simulink model "update_perfil_obstaculos_test"  (R2019a)
settings: Solver=VariableStepAuto  StartTime=0.0  StopTime=10  RelTol=1e-3
undefined symbols (not defined in the file): H_c, x_t_max_oper, x_t_min_oper, y_h_min_oper
libraries: simulink x1
settings Model: Creator=Facundo  LastModifiedBy=Facundo

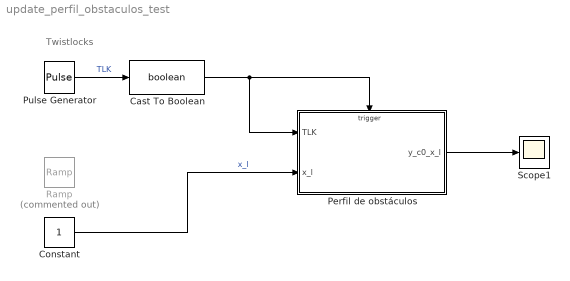
== system update_perfil_obstaculos_test ==
  note: Twistlocks
  Cast To Boolean : DataTypeConversion  OutDataTypeStr=boolean
  Constant : Constant
  Perfil de obstáculos : Subsystem
  Pulse Generator : DiscretePulseGenerator  PulseType=Time based  Period=5  PulseWidth=25  PhaseDelay=2
  Ramp : simulink/Sources/Ramp  Commented=on  slope=1  start=0  InitialOutput=-10
  Scope1 : Scope
  wires:
  Pulse Generator/1 -> Cast To Boolean/1  "TLK"
  Cast To Boolean/1 -> Perfil de obstáculos/Trigger, Perfil de obstáculos/1(TLK)
  Perfil de obstáculos/1(y_c0_x_l) -> Scope1/1
  Constant/1 -> Perfil de obstáculos/2(x_l)  "x_l"

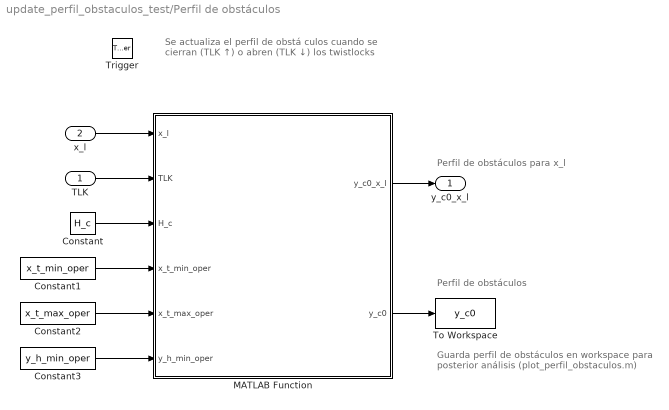
== system update_perfil_obstaculos_test/Perfil de obstáculos ==
  note: Guarda perfil de obstáculos en workspace
      | para posterior análisis (plot_perfil_obstaculos.m)
  note: Perfil de obstáculos para x_l
  note: Se actualiza el perfil de obstá culos cuando
      | se cierran (TLK ↑) o abren (TLK ↓) los twistlocks
  note: Perfil de obstáculos
  TLK : Inport  PortDimensions=1
  x_l : Inport  Port=2  OutDataTypeStr=double  PortDimensions=1
  Trigger : TriggerPort  TriggerType=either  VariantControl=Variant  PortDimensions=1
  Constant : Constant  Value=H_c
  Constant1 : Constant  Value=x_t_min_oper
  Constant2 : Constant  Value=x_t_max_oper
  Constant3 : Constant  Value=y_h_min_oper
  MATLAB Function : MATLAB Function  TreatAsAtomicUnit=on
  To Workspace : ToWorkspace  VariableName=y_c0  SaveFormat=Structure With Time  SampleTime=-1
  y_c0_x_l : Outport  OutDataTypeStr=double  PortDimensions=1  InitialOutput=y_h_min_oper
  wires:
  MATLAB Function/1(y_c0_x_l) -> y_c0_x_l/1
  TLK/1 -> MATLAB Function/2(TLK)
  x_l/1 -> MATLAB Function/1(x_l)
  Constant/1 -> MATLAB Function/3(H_c)
  Constant1/1 -> MATLAB Function/4(x_t_min_oper)
  Constant2/1 -> MATLAB Function/5(x_t_max_oper)
  Constant3/1 -> MATLAB Function/6(y_h_min_oper)
  MATLAB Function/2(y_c0) -> To Workspace/1

== matlab function update_perfil_obstaculos_test/Perfil de obstáculos/MATLAB Function ==
  data: x_l input; y_c0_x_l output; TLK input; H_c input; x_t_min_oper input; x_t_max_oper input; y_h_min_oper input; y_c0 output size=[1, 1651]
function [y_c0_x_l,y_c0] = update_perfil_obstactulos(x_l, TLK, H_c, x_t_min_oper, x_t_max_oper, y_h_min_oper)
    % Actualiza el perfil de obstaculos
    % Entradas:
    % 1) x_l: posición horizontal de la carga 
    % 2) TLK: twistlocks
    % 3) H_c: alto del container estándar
    % 4) x_t_min_oper: límite de operación mínimo de posición horizontal
    % del carro
    % 5) x_t_max_oper: límite de operación máximo de posición horizontal
    % del carro
    % 6) y_h_min_oper: límite de operación mínimo de posición vertical
    % de izaje
    % Salidas:
    % 1) y_c0_x_l: perfil de obstáculo para la posición x_l y tiempo actual
    % 2) y_c0: perfil de obstáculo (vector de altura de obstáculos en
    % función de posición horizontal) para el tiempo actual
    
    persistent y_c0_prev x;
    
    if isempty(y_c0_prev)
        % Inicializar y_c0_prev si es la primera ejecución
        x_min = x_t_min_oper - H_c/2;
        x_max = x_t_max_oper + H_c/2;
        x = x_min:0.05:x_max; % Vector de posiciones horizontales
        y_c0_prev = y_h_min_oper * ones(1, size(x,2)); %Inicializa y_c0_prev con la posición vertical mínima
    end
    
    % Buscar índices donde x está en el rango [x_l ± H_c/2]
    indices = find((x >= (x_l - H_c/2)) & (x <= (x_l + H_c/2)));
    
    % Actualizar y_c0 para dichas posiciones.
    y_c0 = y_c0_prev; % Empieza con valores previos
    
    if (TLK)  % Si se abren los twistlocks (se suelta el contenedor)
        y_c0(indices) = y_c0(indices) + H_c;
    else      % Si se cierran los twistlocks (se agarra el contenedor)
        y_c0(indices) = y_c0(indices) - H_c;
    end
    
    % Buscar índice para x más cercano a x_l
    [~, index] = min(abs(x - x_l));
    y_c0_x_l = y_c0(index); % Actualiza valor de y_c0(x_l)
    
    % Guardar los valores actuales como previos para próxima iteración
    y_c0_prev = y_c0;
end
